simulink model "SINGLE_PHASE_INVERTER_CONTROL"  (R2023a)
settings: Solver=ode45  StartTime=0.0  StopTime=0.1  MaxStep=1e-7  MinStep=1e-8  RelTol=1e-3
libraries: spsIGBTDiodeLib x4, spsSeriesRLCBranchLib x4, spsCurrentMeasurementLib x2, spsDCVoltageSourceLib x1, simulink x1, spsVoltageMeasurementLib x1, sps_lib x1
settings Model: Creator=sudib  LastModifiedBy=sudib

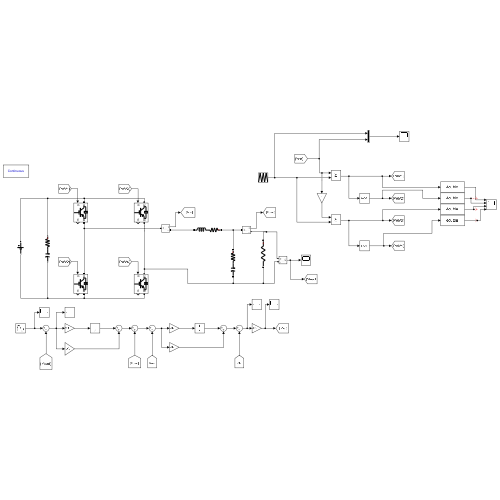
[thumbnail: Simulink's stored preview of the top-level diagram]
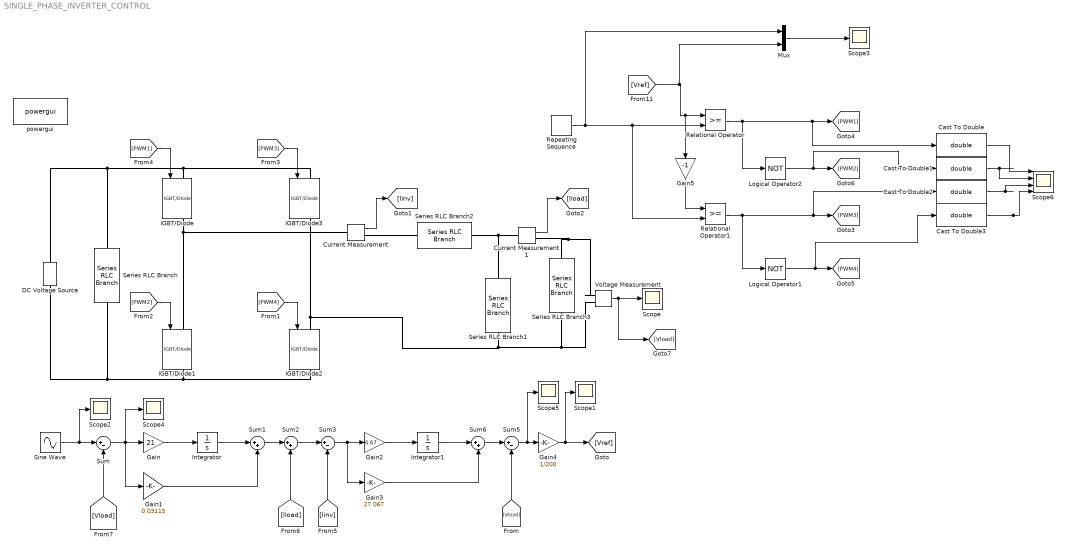
== system SINGLE_PHASE_INVERTER_CONTROL ==
  Cast To Double{,1..3} (4 alike) : DataTypeConversion  OutDataTypeStr=double  SaturateOnIntegerOverflow=off  RndMeth=Floor
  Current Measurement : spsCurrentMeasurementLib/Current Measurement  PhasorSimulation=off  OutputType=Complex  PSBequivalent=0
  Current Measurement1 : spsCurrentMeasurementLib/Current Measurement  PhasorSimulation=off  OutputType=Complex  PSBequivalent=0
  DC Voltage Source : spsDCVoltageSourceLib/DC Voltage Source  Amplitude=300  Measurements=None
  Gain : Gain  Gain=21
  Gain1 : Gain  Gain=0.03115
  Gain2 : Gain  Gain=6.67
  Gain3 : Gain  Gain=27.067
  Gain4 : Gain  Gain=1/200
  Gain5 : Gain  Gain=-1
  IGBT/Diode{,1..3} (4 alike) : spsIGBTDiodeLib/IGBT//Diode  Ron=1e-3  Rs=1e5  Cs=inf  Measurements=on
  Integrator : Integrator
  Integrator1 : Integrator
  Logical Operator1 : Logic  Operator=NOT  AllPortsSameDT=off  OutDataTypeStr=boolean
  Logical Operator2 : Logic  Operator=NOT  AllPortsSameDT=off  OutDataTypeStr=boolean
  Mux : Mux  Inputs=2
  Relational Operator : RelationalOperator  OutDataTypeStr=boolean  RndMeth=Simplest  InputSameDT=off
  Relational Operator1 : RelationalOperator  OutDataTypeStr=boolean  RndMeth=Simplest  InputSameDT=off
  Repeating Sequence : simulink/Sources/Repeating Sequence  rep_seq_t=[0 0.00005 0.0001]  rep_seq_y=[-0.4 0.4 -0.4]
  Scope{,1..5} (6 alike) : Scope
  Scope6 : Scope  NumInputPorts=4
  Series RLC Branch : spsSeriesRLCBranchLib/Series RLC Branch  LConnTagsString=__new0  RConnTagsString=__new0  BranchType=RC  Resistance=0.0042  Inductance=0  SetiL0=off  InitialCurrent=0  Capacitance=500e-6  Setx0=off  InitialVoltage=0  Measurements=None
  Series RLC Branch1 : spsSeriesRLCBranchLib/Series RLC Branch  LConnTagsString=__new0  RConnTagsString=__new0  BranchType=RC  Resistance=0.0042  Inductance=0  SetiL0=off  InitialCurrent=0  Capacitance=6.23e-6  Setx0=off  InitialVoltage=0  Measurements=None
  Series RLC Branch2 : spsSeriesRLCBranchLib/Series RLC Branch  LConnTagsString=__new0  RConnTagsString=__new0  BranchType=RL  Resistance=0.001  Inductance=0.00406  SetiL0=off  InitialCurrent=0  Capacitance=1e-6  Setx0=off  InitialVoltage=0  Measurements=None
  Series RLC Branch3 : spsSeriesRLCBranchLib/Series RLC Branch  LConnTagsString=__new0  RConnTagsString=__new0  BranchType=R  Resistance=100  Inductance=0  SetiL0=off  InitialCurrent=0  Capacitance=1e-6  Setx0=off  InitialVoltage=0  Measurements=None
  Sine Wave : Sin  Amplitude=300  Frequency=314.14  SampleTime=0
  Sum : Sum  Inputs=|+-
  Sum1 : Sum  Inputs=|++
  Sum2 : Sum  Inputs=|++
  Sum3 : Sum  Inputs=|+-
  Sum5 : Sum  Inputs=|+-
  Sum6 : Sum  Inputs=|++
  Voltage Measurement : spsVoltageMeasurementLib/Voltage Measurement  PhasorSimulation=off  OutputType=Complex  PSBequivalent=0
  powergui : sps_lib/powergui  Priority=1  SimulationMode=Continuous  SampleTime=50e-6  frequency=60  Iterations=50  frequencyindice=0  Pbase=100e6  ErrMax=1e-4  UnitsV=kV  UnitsW=MW  buscounter=0  FunctionMessages=off  echomessages=off  EnableUseOfTLC=off  CurrentSourceSwitches=off  DisableSnubberDevices=off  DisableRonSwitches=off  DisableVfSwitches=off  DisplayEquations=off  AutomaticDiscreteSolvers=off  SolverType=Tustin/Backward Euler (TBE)  Interpol=off  ExternalGateDelay=off  methode=off  Ts=100  x0status=blocks  SPID=on  SwTol=0  HookPort=off  NonlinearTolerance=1e-4  nMaxIteration=100  ContinueOnMaxIteration=off  RestoreLinks=warning  ResistiveCurrentMeasurement=off  Frange=[0:2:500]  Ylog=off  Xlog=on  ShowGrid=off  save=off  variable=ZData  structure=0  ZoomFFT=off  StartTime=0.0  cycles=1  DisplayStyle=1  fundamental=60  FreqAxis=off  MaxFrequency=1000  frequencyindicesteady=1  RmsSteady=1  display=off
  wires:
  Current Measurement1/1 -> [Iload]
  Current Measurement/1 -> [Iinv]
  Sum/1 -> Gain1/1, Scope4/1, Gain/1
  Gain/1 -> Integrator/1
  Integrator/1 -> Sum1/1
  Gain1/1 -> Sum1/2
  Sum1/1 -> Sum2/1
  Sum2/1 -> Sum3/1
  Gain2/1 -> Integrator1/1
  Gain3/1 -> Sum6/2
  Integrator1/1 -> Sum6/1
  Sum3/1 -> Gain3/1, Gain2/1
  Sum6/1 -> Sum5/1
  Sum5/1 -> Scope5/1, Gain4/1
  Gain4/1 -> Scope1/1, [Vref]
  [PWM2] -> IGBT/Diode1/1
  [PWM4] -> IGBT/Diode2/1
  [PWM3] -> IGBT/Diode3/1
  [PWM1] -> IGBT/Diode/1
  Sine Wave/1 -> Scope2/1, Sum/1
  [Vload] -> Sum5/2
  [Iinv] -> Sum3/2
  [Iload] -> Sum2/2
  [Vload] -> Sum/2
  [Vref] -> Mux/2, Relational Operator/1, Gain5/1
  Gain5/1 -> Relational Operator1/1
  Relational Operator1/1 -> Logical Operator1/1, Cast To Double2/1, [PWM3]
  Relational Operator/1 -> Cast To Double/1, [PWM1], Logical Operator2/1
  Logical Operator1/1 -> Cast To Double3/1, [PWM4]
  Logical Operator2/1 -> Cast To Double1/1, [PWM2]
  Voltage Measurement/1 -> [Vload], Scope/1
  Repeating Sequence/1 -> Mux/1, Relational Operator1/2, Relational Operator/2
  Mux/1 -> Scope3/1
  Cast To Double3/1 -> Scope6/4
  Cast To Double2/1 -> Scope6/3
  Cast To Double1/1 -> Scope6/2
  Cast To Double/1 -> Scope6/1
  connections:
  DC Voltage Source/RConn1 -- Series RLC Branch/LConn1 -- IGBT/Diode3/LConn1 -- IGBT/Diode/LConn1
  DC Voltage Source/LConn1 -- Series RLC Branch/RConn1 -- IGBT/Diode2/RConn1 -- IGBT/Diode1/RConn1
  IGBT/Diode3/RConn1 -- Voltage Measurement/LConn2 -- Series RLC Branch3/RConn1 -- Series RLC Branch1/RConn1 -- IGBT/Diode2/LConn1
  IGBT/Diode/RConn1 -- IGBT/Diode1/LConn1 -- Current Measurement/LConn1
  Series RLC Branch2/RConn1 -- Current Measurement/RConn1
  Series RLC Branch2/LConn1 -- Current Measurement1/LConn1 -- Series RLC Branch1/LConn1
  Current Measurement1/RConn1 -- Voltage Measurement/LConn1 -- Series RLC Branch3/LConn1
